simulink model "Problem2"  (R2020b)
settings: Solver=VariableStepAuto  StartTime=0.0  StopTime=100.0  RelTol=1e-3
values from neighbouring files (symbols this model uses):
  b = 50    [Dummy_Input.m]
  k1 = 50    [Dummy_Input.m]
  k2 = 300    [Dummy_Input.m]
  m1 = 500    [Dummy_Input.m]
  m2 = 50    [Dummy_Input.m]
settings Model: Creator=Shirish  LastModifiedBy=Shirish
settings DataIOCC: LoadExternalInput=on  SaveOutput=off  SaveTime=off

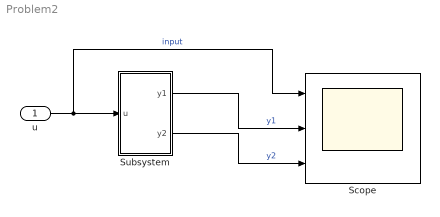
== system Problem2 ==
  u : Inport
  Scope : Scope  NumInputPorts=3
  Subsystem : Subsystem
  wires:
  u/1 -> Scope/1, Subsystem/1(u)  "input"
  Subsystem/1(y1) -> Scope/2  "y1"
  Subsystem/2(y2) -> Scope/3  "y2"

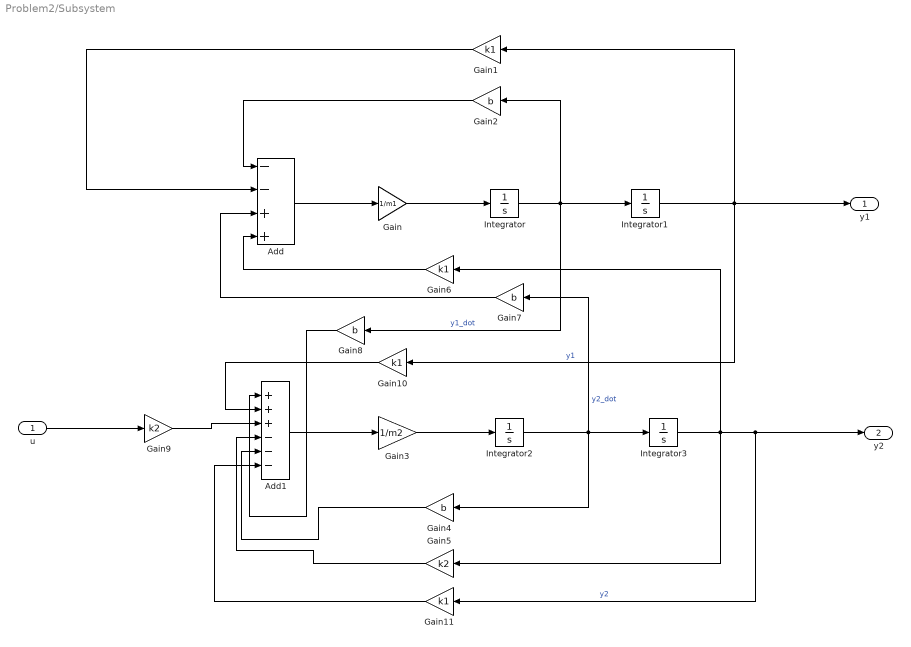
== system Problem2/Subsystem ==
  u : Inport
  Add : Sum  Inputs=--++
  Add1 : Sum  Inputs=+++---
  Gain : Gain  Gain=1/m1
  Gain{1,6,10..11} (4 alike) : Gain  Gain=k1
  Gain{2,4,7..8} (4 alike) : Gain  Gain=b
  Gain3 : Gain  Gain=1/m2
  Gain5 : Gain  Gain=k2
  Gain9 : Gain  Gain=k2
  Integrator{,1..3} (4 alike) : Integrator
  y1 : Outport
  y2 : Outport  Port=2
  wires:
  Integrator1/1 -> Gain1/1, y1/1, Gain10/1  "y1"
  Integrator/1 -> Gain2/1, Integrator1/1, Gain8/1  "y1_dot"
  Gain1/1 -> Add/2
  Add/1 -> Gain/1
  u/1 -> Gain9/1
  Integrator3/1 -> Gain6/1, y2/1, Gain11/1, Gain5/1  "y2"
  Add1/1 -> Gain3/1
  Gain11/1 -> Add1/6
  Integrator2/1 -> Gain7/1, Integrator3/1, Gain4/1  "y2_dot"
  Gain4/1 -> Add1/5
  Gain/1 -> Integrator/1
  Gain2/1 -> Add/1
  Gain8/1 -> Add1/1
  Gain7/1 -> Add/3
  Gain6/1 -> Add/4
  Gain9/1 -> Add1/3
  Gain3/1 -> Integrator2/1
  Gain10/1 -> Add1/2
  Gain5/1 -> Add1/4
